simulink model "DMP_model"  (R2022a)
settings: Solver=ode4  StartTime=0.0  StopTime=during  FixedStep=0.01  RelTol=1e-3
values from neighbouring files (symbols this model uses):
  alphaz = params.alphaz    [get_weights.m]    (also in plot_simu.m = 30)
  K = params.K    [get_weights.m]    (also in plot_simu.m = 10)
  N = params.N    [get_weights.m]    (also in output_dynamical_system.m = (L-2)/2; plot_simu.m = 20)
  w0 = params.w0    [get_weights.m]    (also in plot_simu.m = [pi;2*pi;8.17;10*pi;44])
  yita = params.yita    [get_weights.m]    (also in plot_simu.m = 4)
libraries: dsparch4 x3, simulink x3
settings Model: Creator=STAN  LastModifiedBy=111
settings DataIOCC: ReturnWorkspaceOutputs=off
settings DebuggingCC: UnconnectedInputMsg=warning  UnconnectedOutputMsg=warning  UnconnectedLineMsg=warning
settings RTWCC: DLArmComputeVersion=19.05

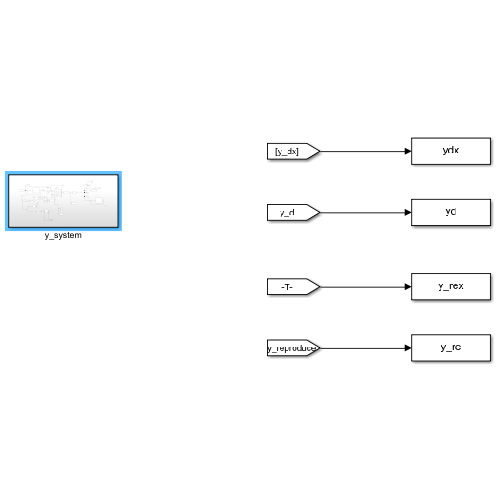
[thumbnail: Simulink's stored preview of the top-level diagram]
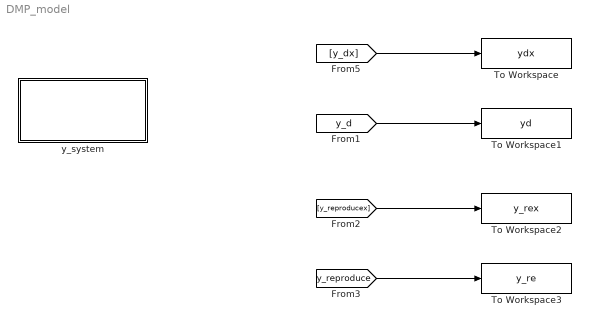
== system DMP_model ==
  To Workspace : ToWorkspace  VariableName=ydx  SaveFormat=Timeseries  SampleTime=-1
  To Workspace1 : ToWorkspace  VariableName=yd  SaveFormat=Timeseries  SampleTime=-1
  To Workspace2 : ToWorkspace  VariableName=y_rex  SaveFormat=Timeseries  SampleTime=-1
  To Workspace3 : ToWorkspace  VariableName=y_re  SaveFormat=Timeseries  SampleTime=-1
  y_system : Subsystem
  wires:
  [y_dx] -> To Workspace/1
  [y_d] -> To Workspace1/1
  [y_reproducex] -> To Workspace2/1
  [y_reproduce] -> To Workspace3/1

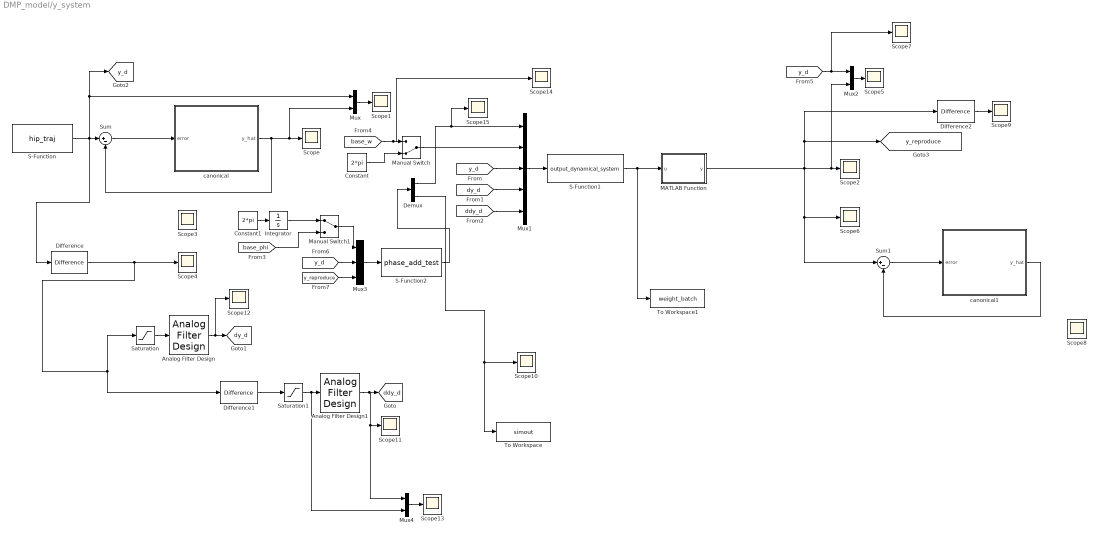
== system DMP_model/y_system ==
  Analog Filter Design : dsparch4/Analog Filter Design  method=Butterworth  filttype=Lowpass  N=3  Wlo=2*pi*20  Whi=80  Rp=2  Rs=40
  Analog Filter Design1 : dsparch4/Analog Filter Design  method=Butterworth  filttype=Lowpass  N=3  Wlo=2*pi*20  Whi=80  Rp=2  Rs=40
  Constant : Constant  Value=2*pi
  Constant1 : Constant  Value=2*pi
  Demux : Demux  Outputs=2
  Difference : simulink/Discrete/Difference  ICPrevInput=0.0  OutMin=[]  OutMax=[]  OutDataType=fixdt(1, 16)  OutScaling=2^-10  DoSatur=off
  Difference1 : simulink/Discrete/Difference  ICPrevInput=0.0  OutMin=[]  OutMax=[]  OutDataType=fixdt(1, 16)  OutScaling=2^-10  DoSatur=off
  Difference2 : simulink/Discrete/Difference  ICPrevInput=0.0  OutMin=[]  OutMax=[]  OutDataType=fixdt(1, 16)  OutScaling=2^-10  DoSatur=off
  Integrator : Integrator
  MATLAB Function : MATLAB Function  TreatAsAtomicUnit=on
  Manual Switch : ManualSwitch  CurrentSetting=0
  Manual Switch1 : ManualSwitch
  Mux : Mux  Inputs=2
  Mux1 : Mux  Inputs=5
  Mux2 : Mux  Inputs=2
  Mux3 : Mux  Inputs=3
  Mux4 : Mux  Inputs=2
  S-Function : S-Function  FunctionName=hip_traj  Parameters=Traj_demo  SFunctionDeploymentMode=off  EnableBusSupport=off
  S-Function1 : S-Function  FunctionName=output_dynamical_system  Parameters=alphaz,N  SFunctionDeploymentMode=off  EnableBusSupport=off
  S-Function2 : S-Function  FunctionName=phase_add_test  SFunctionDeploymentMode=off  EnableBusSupport=off
  Saturation : Saturate  UpperLimit=5  LowerLimit=-5
  Saturation1 : Saturate  UpperLimit=5  LowerLimit=-5
  Scope{,1..15} (16 alike) : Scope
  Sum : Sum  Inputs=|+-
  Sum1 : Sum  Inputs=|+-
  To Workspace : ToWorkspace  VariableName=simout  SaveFormat=Timeseries  SampleTime=-1
  To Workspace1 : ToWorkspace  VariableName=weight_batch  SaveFormat=Timeseries  SampleTime=-1
  canonical : Subsystem
  canonical1 : Subsystem
  tag scope: ddy_d=global, dy_d=global, y_d=global, y_reproduce=global
  wires:
  Sum/1 -> canonical/1(error)
  [y_d] -> Mux1/3
  canonical/1(y_hat) -> Mux/2, Scope/1, Sum/2
  Mux/1 -> Scope1/1
  S-Function/1 -> Difference/1, [y_d], Mux/1, Sum/1
  [ddy_d] -> Mux1/5
  [y_d] -> Scope7/1, Mux2/1
  canonical1/1(y_hat) -> Sum1/2
  MATLAB Function/1(y) -> Sum1/1, Scope6/1, Difference2/1, [y_reproduce], Mux2/2, Scope2/1
  Sum1/1 -> canonical1/1(error)
  Mux2/1 -> Scope5/1
  [dy_d] -> Mux1/4
  Mux1/1 -> S-Function1/1
  Mux3/1 -> S-Function2/1
  [y_d] -> Mux3/2
  [y_reproduce] -> Mux3/3
  S-Function2/1 -> Demux/1
  Demux/1 -> Scope15/1, Mux1/1
  Demux/2 -> To Workspace/1, Scope10/1
  Difference2/1 -> Scope9/1
  Difference/1 -> Scope4/1, Difference1/1, Saturation/1
  Difference1/1 -> Saturation1/1
  Saturation1/1 -> Mux4/2, Analog Filter Design1/1
  Saturation/1 -> Analog Filter Design/1
  Analog Filter Design1/1 -> Mux4/1, Scope11/1, [ddy_d]
  Analog Filter Design/1 -> Scope12/1, [dy_d]
  Mux4/1 -> Scope13/1
  Manual Switch/1 -> Mux1/2
  [base_w] -> Scope14/1, Manual Switch/1
  Constant/1 -> Manual Switch/2
  Constant1/1 -> Integrator/1
  Manual Switch1/1 -> Mux3/1
  Integrator/1 -> Manual Switch1/1
  [base_phi] -> Manual Switch1/2
  S-Function1/1 -> MATLAB Function/1(u), To Workspace1/1

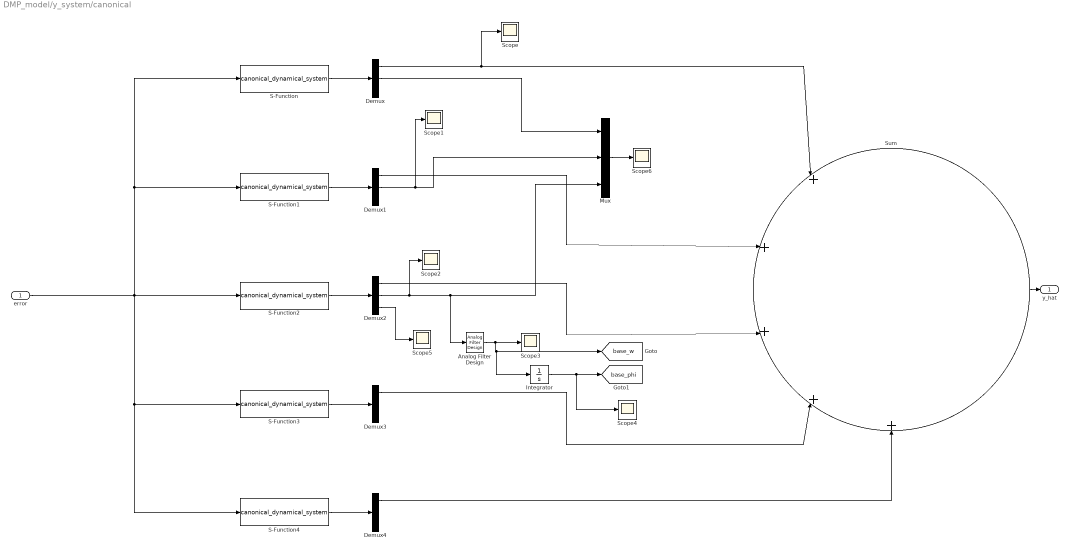
== system DMP_model/y_system/canonical ==
  error : Inport
  Analog Filter Design : dsparch4/Analog Filter Design  method=Butterworth  filttype=Lowpass  N=3  Wlo=2*pi*0.1  Whi=80  Rp=2  Rs=40
  Demux{,1..4} (5 alike) : Demux  Outputs=3
  Integrator : Integrator
  Mux : Mux  Inputs=3
  S-Function : S-Function  FunctionName=canonical_dynamical_system  Parameters=K,yita,w0(1)  SFunctionDeploymentMode=off  EnableBusSupport=off
  S-Function1 : S-Function  FunctionName=canonical_dynamical_system  Parameters=K,yita,w0(2)  SFunctionDeploymentMode=off  EnableBusSupport=off
  S-Function2 : S-Function  FunctionName=canonical_dynamical_system  Parameters=K,yita,w0(3)  SFunctionDeploymentMode=off  EnableBusSupport=off
  S-Function3 : S-Function  FunctionName=canonical_dynamical_system  Parameters=K,yita,w0(4)  SFunctionDeploymentMode=off  EnableBusSupport=off
  S-Function4 : S-Function  FunctionName=canonical_dynamical_system  Parameters=K,yita,w0(5)  SFunctionDeploymentMode=off  EnableBusSupport=off
  Scope{,1..6} (7 alike) : Scope
  Sum : Sum  Inputs=|+++++
  y_hat : Outport
  tag scope: base_phi=global, base_w=global
  wires:
  S-Function3/1 -> Demux3/1
  S-Function4/1 -> Demux4/1
  S-Function/1 -> Demux/1
  S-Function1/1 -> Demux1/1
  Demux1/1 -> Sum/2
  Demux3/1 -> Sum/4
  S-Function2/1 -> Demux2/1
  Demux/1 -> Scope/1, Sum/1
  Demux2/1 -> Sum/3
  Demux4/1 -> Sum/5
  Sum/1 -> y_hat/1
  error/1 -> S-Function4/1, S-Function3/1, S-Function2/1, S-Function1/1, S-Function/1
  Demux1/2 -> Scope1/1, Mux/2
  Demux2/2 -> Scope2/1, Mux/3, Analog Filter Design/1
  Demux/2 -> Mux/1
  Mux/1 -> Scope6/1
  Analog Filter Design/1 -> Integrator/1, [base_w], Scope3/1
  Integrator/1 -> Scope4/1, [base_phi]
  Demux2/3 -> Scope5/1

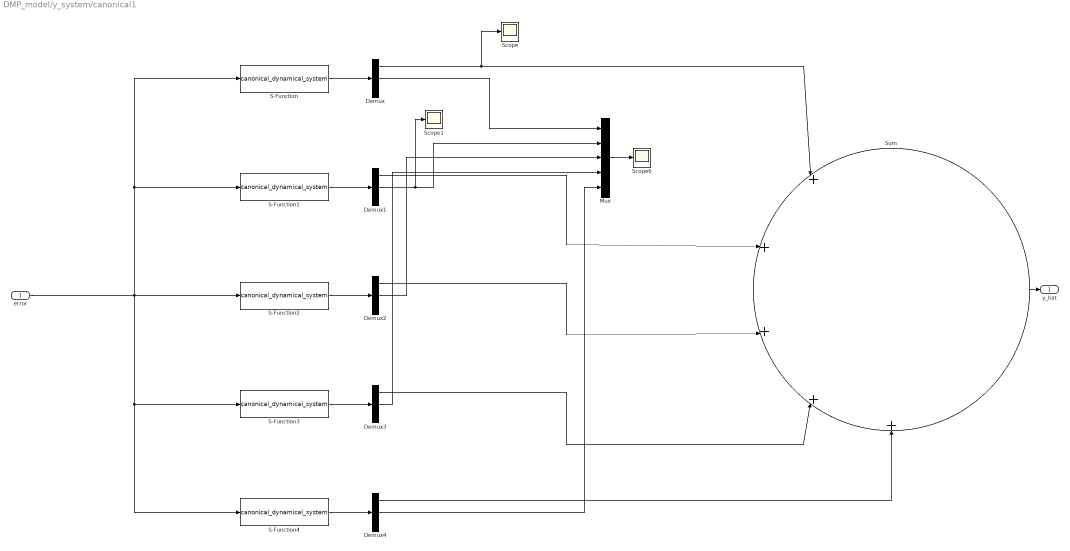
== system DMP_model/y_system/canonical1 ==
  error : Inport
  Demux{,1..4} (5 alike) : Demux  Outputs=3
  Mux : Mux  Inputs=5
  S-Function : S-Function  FunctionName=canonical_dynamical_system  Parameters=K,yita,w0(1)  SFunctionDeploymentMode=off  EnableBusSupport=off
  S-Function1 : S-Function  FunctionName=canonical_dynamical_system  Parameters=K,yita,w0(2)  SFunctionDeploymentMode=off  EnableBusSupport=off
  S-Function2 : S-Function  FunctionName=canonical_dynamical_system  Parameters=K,yita,w0(3)  SFunctionDeploymentMode=off  EnableBusSupport=off
  S-Function3 : S-Function  FunctionName=canonical_dynamical_system  Parameters=K,yita,w0(4)  SFunctionDeploymentMode=off  EnableBusSupport=off
  S-Function4 : S-Function  FunctionName=canonical_dynamical_system  Parameters=K,yita,w0(5)  SFunctionDeploymentMode=off  EnableBusSupport=off
  Scope : Scope
  Scope1 : Scope
  Scope6 : Scope
  Sum : Sum  Inputs=|+++++
  y_hat : Outport
  wires:
  S-Function3/1 -> Demux3/1
  S-Function4/1 -> Demux4/1
  S-Function/1 -> Demux/1
  S-Function1/1 -> Demux1/1
  Demux1/1 -> Sum/2
  Demux3/1 -> Sum/4
  S-Function2/1 -> Demux2/1
  Demux/1 -> Scope/1, Sum/1
  Demux2/1 -> Sum/3
  Demux4/1 -> Sum/5
  Sum/1 -> y_hat/1
  error/1 -> S-Function4/1, S-Function3/1, S-Function2/1, S-Function1/1, S-Function/1
  Demux3/2 -> Mux/4
  Demux1/2 -> Scope1/1, Mux/2
  Demux2/2 -> Mux/3
  Demux4/2 -> Mux/5
  Demux/2 -> Mux/1
  Mux/1 -> Scope6/1

== matlab function DMP_model/y_system/MATLAB Function ==
  data: u input; y output
function y = tfer(u)

y = u(1);
